simulink model "Subsystem1"  (R2020b)
settings: Solver=FixedStepAuto  StartTime=0.0  StopTime=10.0  FixedStep=0.1  RelTol=1e-3
settings Model: Creator=samar  LastModifiedBy=samar
settings DataIOCC: SaveOutput=off  SaveTime=off

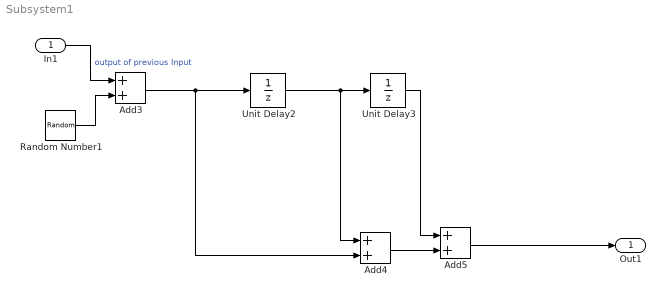
== system Subsystem1 ==
  In1 : Inport  OutDataTypeStr=double  PortDimensions=1  SampleTime=[0.10000000000000001,0]
  Add3 : Sum
  Add4 : Sum
  Add5 : Sum
  Random Number1 : RandomNumber  Mean=1  Variance=0.01  SampleTime=0.1
  Unit Delay2 : UnitDelay  SampleTime=-1  HasFrameUpgradeWarning=on
  Unit Delay3 : UnitDelay  SampleTime=-1  HasFrameUpgradeWarning=on
  Out1 : Outport  OutDataTypeStr=double  PortDimensions=1  SampleTime=[0.10000000000000001,0]
  wires:
  In1/1 -> Add3/1  "output of previous Input"
  Add3/1 -> Unit Delay2/1, Add4/2
  Add5/1 -> Out1/1
  Unit Delay2/1 -> Unit Delay3/1, Add4/1
  Random Number1/1 -> Add3/2
  Unit Delay3/1 -> Add5/1
  Add4/1 -> Add5/2
